simulink model "AM2"  (R2020b)
settings: Solver=VariableStepDiscrete  StartTime=0.0  StopTime=3  MaxStep=1/400  RelTol=1e-3
settings Model: Creator=seojoon  LastModifiedBy=seojoon

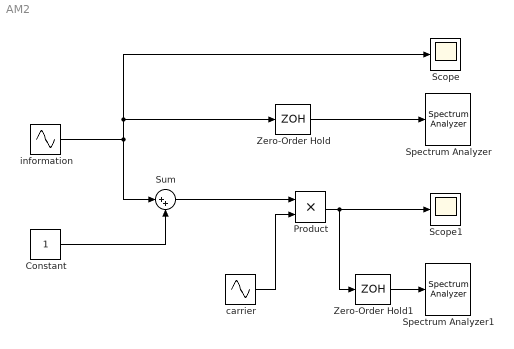
== system AM2 ==
  Constant : Constant
  Product : Product
  Scope : Scope
  Scope1 : Scope
  Spectrum Analyzer : SpectrumAnalyzer
  Spectrum Analyzer1 : SpectrumAnalyzer
  Sum : Sum  Inputs=|++
  Zero-Order Hold : ZeroOrderHold  SampleTime=1/1000
  Zero-Order Hold1 : ZeroOrderHold  SampleTime=1/1000
  carrier : Sin  Frequency=2*pi*50  Phase=pi/2  SampleTime=0
  information : Sin  Amplitude=2  Frequency=2*pi*3  SampleTime=0
  wires:
  information/1 -> Sum/1, Scope/1, Zero-Order Hold/1
  Constant/1 -> Sum/2
  Sum/1 -> Product/1
  carrier/1 -> Product/2
  Product/1 -> Zero-Order Hold1/1, Scope1/1
  Zero-Order Hold/1 -> Spectrum Analyzer/1
  Zero-Order Hold1/1 -> Spectrum Analyzer1/1
